simulink model "a1_ex2_sim3"  (R2023a)
settings: Solver=FixedStepAuto  StartTime=0.0  StopTime=30  FixedStep=Ts  RelTol=1e-3
InitFcn:
  | a1_ex2_sim_init
values from neighbouring files (symbols this model uses):
  filter_coeff_bp = firpm(n_bp,fo_bp,ao_bp,w_bp)    [a1_ex2_sim_init.m]
  filter_coeff_lp = firpm(n_lp,fo_lp,ao_lp,w_lp)    [a1_ex2_sim_init.m]
  R = [cos(theta) -sin(theta) 0 ... (first row only)    [a1_ex2_sim_init.m]
  rate_limit_falling = -2    [a1_ex2_sim_init.m]
  rate_limit_rising = 2    [a1_ex2_sim_init.m]
  th1_biceps_left = 0.09    [a1_ex2_sim_init.m]
  th1_biceps_right = 0.09    [a1_ex2_sim_init.m]
  th1_trapezius_left = 0.055    [a1_ex2_sim_init.m]
  th1_trapezius_right = 0.08    [a1_ex2_sim_init.m]
  Ts = 1e-3    (= 0.001)    [a1_ex2_sim_init.m]
undefined symbols (not defined in the file or in its folder): DiscIntNeverNeededParam
libraries: spsEdgeDetectorLib x4, vrlib x1
settings Model: Creator=davide  LastModifiedBy=davide

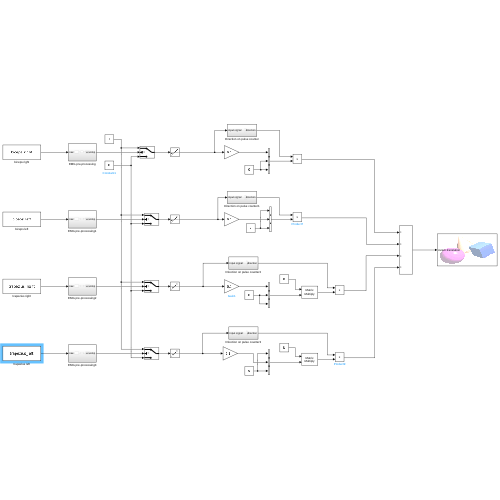
[thumbnail: Simulink's stored preview of the top-level diagram]
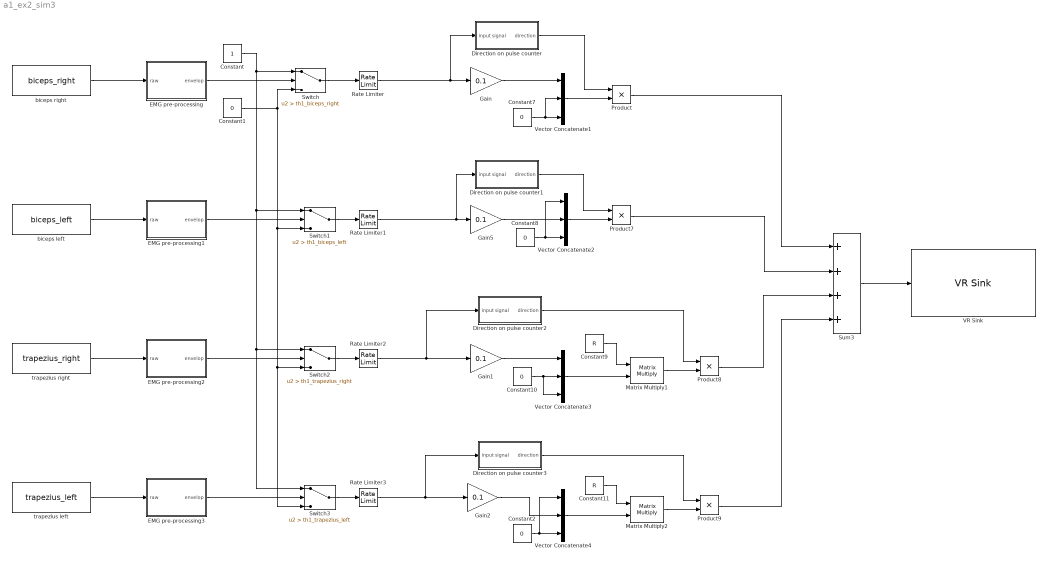
== system a1_ex2_sim3 ==
  Constant : Constant
  Constant{1..2,7..8,10} (5 alike) : Constant  Value=0
  Constant11 : Constant  Value=R  VectorParams1D=off
  Constant9 : Constant  Value=R  VectorParams1D=off
  Direction on pulse counter : Subsystem
  Direction on pulse counter1 : Subsystem
  Direction on pulse counter2 : Subsystem
  Direction on pulse counter3 : Subsystem
  EMG pre-processing : Subsystem
  EMG pre-processing1 : Subsystem
  EMG pre-processing2 : Subsystem
  EMG pre-processing3 : Subsystem
  Gain{,1..2,5} (4 alike) : Gain  Gain=0.1
  Matrix Multiply1 : Product  Multiplication=Matrix(*)
  Matrix Multiply2 : Product  Multiplication=Matrix(*)
  Product{,7..9} (4 alike) : Product
  Rate Limiter{,1..3} (4 alike) : RateLimiter  RisingSlewLimit=rate_limit_rising  FallingSlewLimit=rate_limit_falling  SampleTimeMode=inherited
  Sum3 : Sum  Inputs=++++
  Switch : Switch  Criteria=u2 > Threshold  Threshold=th1_biceps_right  SaturateOnIntegerOverflow=off  InputSameDT=off
  Switch1 : Switch  Criteria=u2 > Threshold  Threshold=th1_biceps_left  SaturateOnIntegerOverflow=off  InputSameDT=off
  Switch2 : Switch  Criteria=u2 > Threshold  Threshold=th1_trapezius_right  SaturateOnIntegerOverflow=off  InputSameDT=off
  Switch3 : Switch  Criteria=u2 > Threshold  Threshold=th1_trapezius_left  SaturateOnIntegerOverflow=off  InputSameDT=off
  VR Sink : vrlib/VR Sink  InstantiateOnLoad=on  SampleTime=0.1  ViewEnable=on  RemoteChange=off  RemoteView=off  FieldsWritten=cursor.translation.3.1.1.double  WorldFileName=es2_emg/8_palline_color.wrl  AutoView=off  VideoDimensions=[]  AllowVariableSize=off  FigureProperties="{'Position', 'Name', 'Viewpoint', 'CameraBound', 'CameraDirection', 'CameraPosition', 'CameraUpVector', 'ZoomFactor', 'Antialiasing', 'Headlight', 'Lighting', 'NavPanel', 'Sound', 'StatusBar', 'Stereo3D', 'Stereo3DCameraOffset', 'Stereo3DHIT', 'ToolBar', 'Textures', 'Transparency', 'Triad', 'Wireframe', 'NavZones', 'NavMode', 'NavSpeed', 'CaptureFileFormat', 'CaptureFileName', 'Record2DCompressMethod', 'Record2DCompressQuality', 'Record2D', 'Record2DFileName', 'Record2DFPS'; [7.5000000000000000e+01   1.1800000000000000e+02   5.6600000000000000e+02   3.5700000000000000e+02], '', '_untitled_1', 'on', [0.0000000000000000e+00   0.0000000000000000e+00  -1.0000000000000000e+00], [0.0000000000000000e+00   0.0000000000000000e+00   0.0000000000000000e+00], [0.0000000000000000e+00   1.0000000000000000e+00   0.0000000000000000e+00], [1.0000000000000000e+00], 'on', 'on', 'on', 'halfbar', 'on', 'on', 'off', [1.0000000149011612e-01], [0.0000000000000000e+00], 'on', 'on', 'on', 'none', 'off', 'off', 'fly', 'normal', 'tif', '%f_anim_%n.tif', 'auto', [7.5000000000000000e+01], 'off', '%f_anim_%n.avi', 'auto'}"
  Vector Concatenate{1..4} (4 alike) : Concatenate  NumInputs=3
  biceps left : FromWorkspace  VariableName=biceps_left  OutDataTypeStr=double  SampleTime=Ts
  biceps right : FromWorkspace  VariableName=biceps_right  OutDataTypeStr=double  SampleTime=Ts
  trapezius left : FromWorkspace  VariableName=trapezius_left  OutDataTypeStr=double  SampleTime=Ts
  trapezius right : FromWorkspace  VariableName=trapezius_right  OutDataTypeStr=double  SampleTime=Ts
  wires:
  biceps right/1 -> EMG pre-processing/1(raw)
  biceps left/1 -> EMG pre-processing1/1(raw)
  trapezius right/1 -> EMG pre-processing2/1(raw)
  trapezius left/1 -> EMG pre-processing3/1(raw)
  Constant/1 -> Switch/1, Switch1/1, Switch2/1, Switch3/1
  Constant1/1 -> Switch/3, Switch1/3, Switch2/3, Switch3/3
  Switch1/1 -> Rate Limiter1/1
  EMG pre-processing2/1(envelop) -> Switch2/2
  Switch2/1 -> Rate Limiter2/1
  Switch3/1 -> Rate Limiter3/1
  EMG pre-processing3/1(envelop) -> Switch3/2
  Rate Limiter3/1 -> Direction on pulse counter3/1(input signal), Gain2/1
  Rate Limiter/1 -> Direction on pulse counter/1(input signal), Gain/1
  Rate Limiter2/1 -> Gain1/1, Direction on pulse counter2/1(input signal)
  EMG pre-processing/1(envelop) -> Switch/2
  EMG pre-processing1/1(envelop) -> Switch1/2
  Switch/1 -> Rate Limiter/1
  Rate Limiter1/1 -> Direction on pulse counter1/1(input signal), Gain5/1
  Gain/1 -> Vector Concatenate1/1
  Constant7/1 -> Vector Concatenate1/2, Vector Concatenate1/3
  Vector Concatenate1/1 -> Product/2
  Direction on pulse counter/1(direction) -> Product/1
  Constant8/1 -> Vector Concatenate2/1, Vector Concatenate2/3
  Gain5/1 -> Vector Concatenate2/2
  Direction on pulse counter1/1(direction) -> Product7/1
  Vector Concatenate2/1 -> Product7/2
  Product/1 -> Sum3/1
  Product7/1 -> Sum3/2
  Constant9/1 -> Matrix Multiply1/1
  Constant10/1 -> Vector Concatenate3/3, Vector Concatenate3/2
  Gain1/1 -> Vector Concatenate3/1
  Vector Concatenate3/1 -> Matrix Multiply1/2
  Direction on pulse counter2/1(direction) -> Product8/1
  Matrix Multiply1/1 -> Product8/2
  Direction on pulse counter3/1(direction) -> Product9/1
  Matrix Multiply2/1 -> Product9/2
  Constant11/1 -> Matrix Multiply2/1
  Constant2/1 -> Vector Concatenate4/1, Vector Concatenate4/3
  Vector Concatenate4/1 -> Matrix Multiply2/2
  Gain2/1 -> Vector Concatenate4/2
  Product8/1 -> Sum3/3
  Product9/1 -> Sum3/4
  Sum3/1 -> VR Sink/1

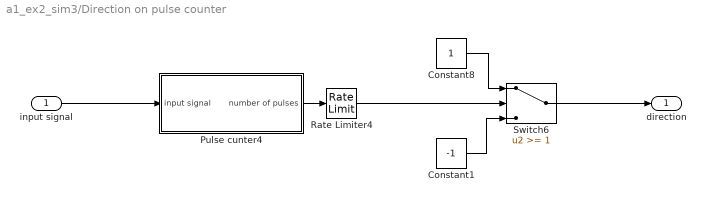
== system a1_ex2_sim3/Direction on pulse counter ==
  input signal : Inport
  Constant1 : Constant  Value=-1  VectorParams1D=off
  Constant8 : Constant  VectorParams1D=off
  Pulse cunter4 : Subsystem
  Rate Limiter4 : RateLimiter  RisingSlewLimit=rate_limit_rising  FallingSlewLimit=rate_limit_falling  SampleTimeMode=inherited
  Switch6 : Switch  Threshold=1  OutDataTypeStr=double  SaturateOnIntegerOverflow=off  InputSameDT=off
  direction : Outport
  wires:
  Pulse cunter4/1(number of pulses) -> Rate Limiter4/1
  Rate Limiter4/1 -> Switch6/2
  Constant1/1 -> Switch6/3
  Constant8/1 -> Switch6/1
  input signal/1 -> Pulse cunter4/1(input signal)
  Switch6/1 -> direction/1

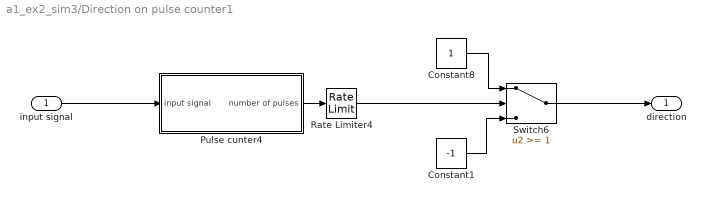
== system a1_ex2_sim3/Direction on pulse counter1 ==
  input signal : Inport
  Constant1 : Constant  Value=-1  VectorParams1D=off
  Constant8 : Constant  VectorParams1D=off
  Pulse cunter4 : Subsystem
  Rate Limiter4 : RateLimiter  RisingSlewLimit=rate_limit_rising  FallingSlewLimit=rate_limit_falling  SampleTimeMode=inherited
  Switch6 : Switch  Threshold=1  OutDataTypeStr=double  SaturateOnIntegerOverflow=off  InputSameDT=off
  direction : Outport
  wires:
  Switch6/1 -> direction/1
  input signal/1 -> Pulse cunter4/1(input signal)
  Constant8/1 -> Switch6/1
  Constant1/1 -> Switch6/3
  Rate Limiter4/1 -> Switch6/2
  Pulse cunter4/1(number of pulses) -> Rate Limiter4/1

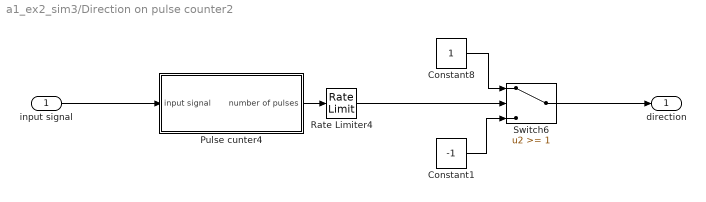
== system a1_ex2_sim3/Direction on pulse counter2 ==
  input signal : Inport
  Constant1 : Constant  Value=-1  VectorParams1D=off
  Constant8 : Constant  VectorParams1D=off
  Pulse cunter4 : Subsystem
  Rate Limiter4 : RateLimiter  RisingSlewLimit=rate_limit_rising  FallingSlewLimit=rate_limit_falling  SampleTimeMode=inherited
  Switch6 : Switch  Threshold=1  OutDataTypeStr=double  SaturateOnIntegerOverflow=off  InputSameDT=off
  direction : Outport
  wires:
  Pulse cunter4/1(number of pulses) -> Rate Limiter4/1
  Rate Limiter4/1 -> Switch6/2
  Constant1/1 -> Switch6/3
  Constant8/1 -> Switch6/1
  input signal/1 -> Pulse cunter4/1(input signal)
  Switch6/1 -> direction/1

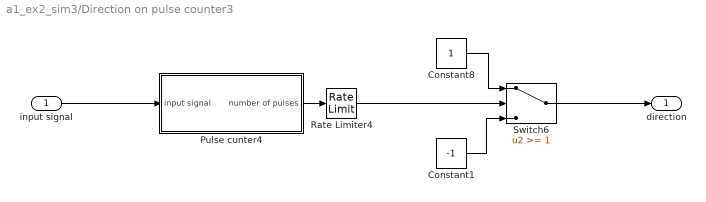
== system a1_ex2_sim3/Direction on pulse counter3 ==
  input signal : Inport
  Constant1 : Constant  Value=-1  VectorParams1D=off
  Constant8 : Constant  VectorParams1D=off
  Pulse cunter4 : Subsystem
  Rate Limiter4 : RateLimiter  RisingSlewLimit=rate_limit_rising  FallingSlewLimit=rate_limit_falling  SampleTimeMode=inherited
  Switch6 : Switch  Threshold=1  OutDataTypeStr=double  SaturateOnIntegerOverflow=off  InputSameDT=off
  direction : Outport
  wires:
  Pulse cunter4/1(number of pulses) -> Rate Limiter4/1
  Rate Limiter4/1 -> Switch6/2
  Constant1/1 -> Switch6/3
  Constant8/1 -> Switch6/1
  input signal/1 -> Pulse cunter4/1(input signal)
  Switch6/1 -> direction/1

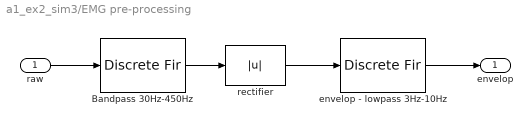
== system a1_ex2_sim3/EMG pre-processing ==
  raw : Inport
  Bandpass 30Hz-450Hz : DiscreteFir  Coefficients=filter_coeff_bp  InputProcessing=Columns as channels (frame based)  SampleTime=Ts
  envelop - lowpass 3Hz-10Hz : DiscreteFir  Coefficients=filter_coeff_lp  InputProcessing=Columns as channels (frame based)  SampleTime=Ts
  rectifier : Abs  SaturateOnIntegerOverflow=off
  envelop : Outport
  wires:
  Bandpass 30Hz-450Hz/1 -> rectifier/1
  rectifier/1 -> envelop - lowpass 3Hz-10Hz/1
  envelop - lowpass 3Hz-10Hz/1 -> envelop/1
  raw/1 -> Bandpass 30Hz-450Hz/1

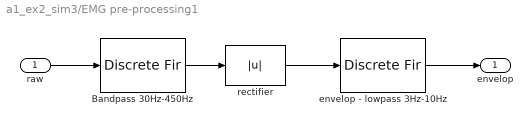
== system a1_ex2_sim3/EMG pre-processing1 ==
  raw : Inport
  Bandpass 30Hz-450Hz : DiscreteFir  Coefficients=filter_coeff_bp  InputProcessing=Columns as channels (frame based)  SampleTime=Ts
  envelop - lowpass 3Hz-10Hz : DiscreteFir  Coefficients=filter_coeff_lp  InputProcessing=Columns as channels (frame based)  SampleTime=Ts
  rectifier : Abs  SaturateOnIntegerOverflow=off
  envelop : Outport
  wires:
  Bandpass 30Hz-450Hz/1 -> rectifier/1
  rectifier/1 -> envelop - lowpass 3Hz-10Hz/1
  envelop - lowpass 3Hz-10Hz/1 -> envelop/1
  raw/1 -> Bandpass 30Hz-450Hz/1

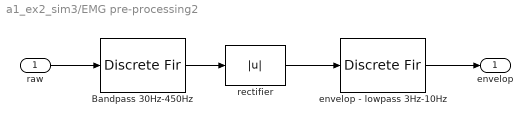
== system a1_ex2_sim3/EMG pre-processing2 ==
  raw : Inport
  Bandpass 30Hz-450Hz : DiscreteFir  Coefficients=filter_coeff_bp  InputProcessing=Columns as channels (frame based)  SampleTime=Ts
  envelop - lowpass 3Hz-10Hz : DiscreteFir  Coefficients=filter_coeff_lp  InputProcessing=Columns as channels (frame based)  SampleTime=Ts
  rectifier : Abs  SaturateOnIntegerOverflow=off
  envelop : Outport
  wires:
  raw/1 -> Bandpass 30Hz-450Hz/1
  envelop - lowpass 3Hz-10Hz/1 -> envelop/1
  rectifier/1 -> envelop - lowpass 3Hz-10Hz/1
  Bandpass 30Hz-450Hz/1 -> rectifier/1

== system a1_ex2_sim3/EMG pre-processing3 ==
  raw : Inport
  Bandpass 30Hz-450Hz : DiscreteFir  Coefficients=filter_coeff_bp  InputProcessing=Columns as channels (frame based)  SampleTime=Ts
  envelop - lowpass 3Hz-10Hz : DiscreteFir  Coefficients=filter_coeff_lp  InputProcessing=Columns as channels (frame based)  SampleTime=Ts
  rectifier : Abs  SaturateOnIntegerOverflow=off
  envelop : Outport
  wires:
  Bandpass 30Hz-450Hz/1 -> rectifier/1
  rectifier/1 -> envelop - lowpass 3Hz-10Hz/1
  envelop - lowpass 3Hz-10Hz/1 -> envelop/1
  raw/1 -> Bandpass 30Hz-450Hz/1

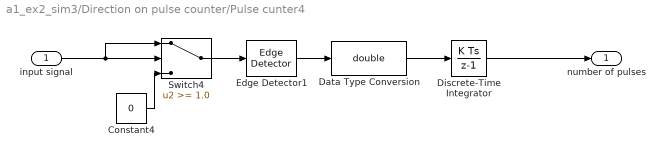
== system a1_ex2_sim3/Direction on pulse counter/Pulse cunter4 ==
  input signal : Inport  SampleTime=Ts
  Constant4 : Constant  Value=0
  Data Type Conversion : DataTypeConversion  OutDataTypeStr=double  SaturateOnIntegerOverflow=off  RndMeth=Floor
  Discrete-Time Integrator : DiscreteIntegrator  gainval=1/Ts  SampleTime=Ts  ICPrevOutput=DiscIntNeverNeededParam  ICPrevScaledInput=DiscIntNeverNeededParam
  Edge Detector1 : spsEdgeDetectorLib/Edge Detector  model=Falling  ic=0  Ts=Ts
      settings: LibrarySourceBlock=sps_lib/Control/Edge Detector
  Switch4 : Switch  Threshold=1.0  SaturateOnIntegerOverflow=off  InputSameDT=off
  number of pulses : Outport
  wires:
  Switch4/1 -> Edge Detector1/1
  Constant4/1 -> Switch4/3
  input signal/1 -> Switch4/1, Switch4/2
  Edge Detector1/1 -> Data Type Conversion/1
  Discrete-Time Integrator/1 -> number of pulses/1
  Data Type Conversion/1 -> Discrete-Time Integrator/1

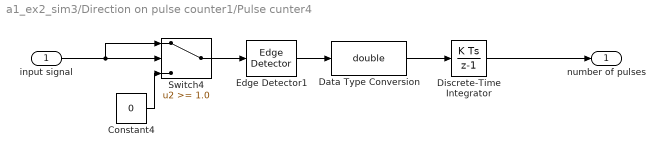
== system a1_ex2_sim3/Direction on pulse counter1/Pulse cunter4 ==
  input signal : Inport  SampleTime=Ts
  Constant4 : Constant  Value=0
  Data Type Conversion : DataTypeConversion  OutDataTypeStr=double  SaturateOnIntegerOverflow=off  RndMeth=Floor
  Discrete-Time Integrator : DiscreteIntegrator  gainval=1/Ts  SampleTime=Ts  ICPrevOutput=DiscIntNeverNeededParam  ICPrevScaledInput=DiscIntNeverNeededParam
  Edge Detector1 : spsEdgeDetectorLib/Edge Detector  model=Falling  ic=0  Ts=Ts
      settings: LibrarySourceBlock=sps_lib/Control/Edge Detector
  Switch4 : Switch  Threshold=1.0  SaturateOnIntegerOverflow=off  InputSameDT=off
  number of pulses : Outport
  wires:
  Data Type Conversion/1 -> Discrete-Time Integrator/1
  Discrete-Time Integrator/1 -> number of pulses/1
  Edge Detector1/1 -> Data Type Conversion/1
  input signal/1 -> Switch4/2, Switch4/1
  Constant4/1 -> Switch4/3
  Switch4/1 -> Edge Detector1/1

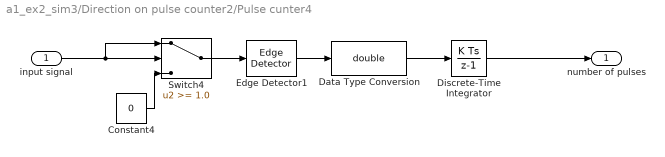
== system a1_ex2_sim3/Direction on pulse counter2/Pulse cunter4 ==
  input signal : Inport  SampleTime=Ts
  Constant4 : Constant  Value=0
  Data Type Conversion : DataTypeConversion  OutDataTypeStr=double  SaturateOnIntegerOverflow=off  RndMeth=Floor
  Discrete-Time Integrator : DiscreteIntegrator  gainval=1/Ts  SampleTime=Ts  ICPrevOutput=DiscIntNeverNeededParam  ICPrevScaledInput=DiscIntNeverNeededParam
  Edge Detector1 : spsEdgeDetectorLib/Edge Detector  model=Falling  ic=0  Ts=Ts
      settings: LibrarySourceBlock=sps_lib/Control/Edge Detector
  Switch4 : Switch  Threshold=1.0  SaturateOnIntegerOverflow=off  InputSameDT=off
  number of pulses : Outport
  wires:
  Switch4/1 -> Edge Detector1/1
  Constant4/1 -> Switch4/3
  input signal/1 -> Switch4/1, Switch4/2
  Edge Detector1/1 -> Data Type Conversion/1
  Discrete-Time Integrator/1 -> number of pulses/1
  Data Type Conversion/1 -> Discrete-Time Integrator/1

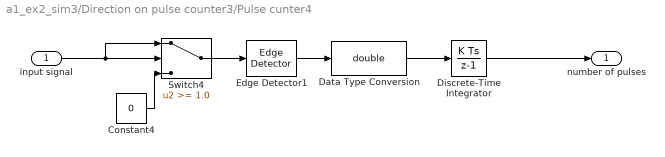
== system a1_ex2_sim3/Direction on pulse counter3/Pulse cunter4 ==
  input signal : Inport  SampleTime=Ts
  Constant4 : Constant  Value=0
  Data Type Conversion : DataTypeConversion  OutDataTypeStr=double  SaturateOnIntegerOverflow=off  RndMeth=Floor
  Discrete-Time Integrator : DiscreteIntegrator  gainval=1/Ts  SampleTime=Ts  ICPrevOutput=DiscIntNeverNeededParam  ICPrevScaledInput=DiscIntNeverNeededParam
  Edge Detector1 : spsEdgeDetectorLib/Edge Detector  model=Falling  ic=0  Ts=Ts
      settings: LibrarySourceBlock=sps_lib/Control/Edge Detector
  Switch4 : Switch  Threshold=1.0  SaturateOnIntegerOverflow=off  InputSameDT=off
  number of pulses : Outport
  wires:
  Switch4/1 -> Edge Detector1/1
  Constant4/1 -> Switch4/3
  input signal/1 -> Switch4/1, Switch4/2
  Edge Detector1/1 -> Data Type Conversion/1
  Discrete-Time Integrator/1 -> number of pulses/1
  Data Type Conversion/1 -> Discrete-Time Integrator/1
